simulink model "CoreLogic"  (R2020a)
settings: Solver=VariableStepAuto  StartTime=0.0  StopTime=10.0  RelTol=1e-3
settings Model: Creator=ANAMIKADUBEY  LastModifiedBy=soumyakantapanda

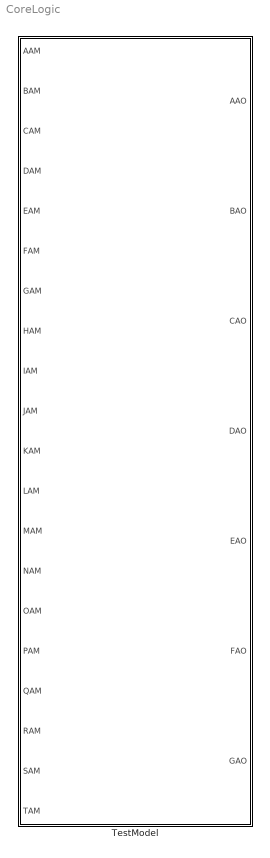
== system CoreLogic ==
  TestModel : Subsystem

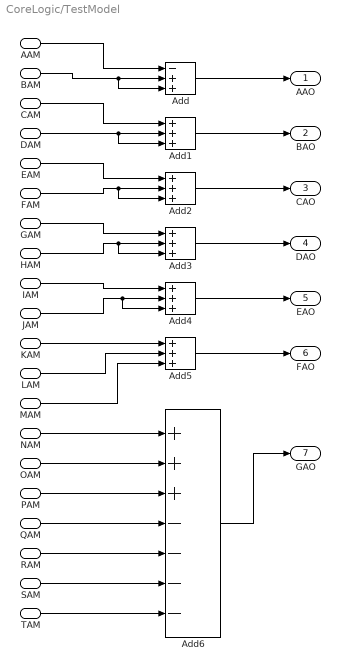
== system CoreLogic/TestModel ==
  AAM : Inport
  BAM : Inport  Port=2
  CAM : Inport  Port=3
  DAM : Inport  Port=4
  EAM : Inport  Port=5
  FAM : Inport  Port=6
  GAM : Inport  Port=7
  HAM : Inport  Port=8
  IAM : Inport  Port=9
  JAM : Inport  Port=10
  KAM : Inport  Port=11
  LAM : Inport  Port=12
  MAM : Inport  Port=13
  NAM : Inport  Port=14
  OAM : Inport  Port=15
  PAM : Inport  Port=16
  QAM : Inport  Port=17
  RAM : Inport  Port=18
  SAM : Inport  Port=19
  TAM : Inport  Port=20
  Add : Sum  Inputs=-++
  Add{1..5} (5 alike) : Sum  Inputs=+++
  Add6 : Sum  Inputs=+++----
  AAO : Outport
  BAO : Outport  Port=2
  CAO : Outport  Port=3
  DAO : Outport  Port=4
  EAO : Outport  Port=5
  FAO : Outport  Port=6
  GAO : Outport  Port=7
  wires:
  Add/1 -> AAO/1
  Add1/1 -> BAO/1
  Add2/1 -> CAO/1
  Add3/1 -> DAO/1
  Add4/1 -> EAO/1
  Add5/1 -> FAO/1
  Add6/1 -> GAO/1
  AAM/1 -> Add/1
  BAM/1 -> Add/3, Add/2
  CAM/1 -> Add1/1
  DAM/1 -> Add1/3, Add1/2
  EAM/1 -> Add2/1
  FAM/1 -> Add2/3, Add2/2
  GAM/1 -> Add3/1
  HAM/1 -> Add3/3, Add3/2
  IAM/1 -> Add4/1
  JAM/1 -> Add4/3, Add4/2
  KAM/1 -> Add5/1
  LAM/1 -> Add5/2
  MAM/1 -> Add5/3
  NAM/1 -> Add6/1
  OAM/1 -> Add6/2
  PAM/1 -> Add6/3
  QAM/1 -> Add6/4
  RAM/1 -> Add6/5
  SAM/1 -> Add6/6
  TAM/1 -> Add6/7
